simulink model "hw2_q3_part_two"  (R2022b)
settings: Solver=ode4  StartTime=0.0  StopTime=10.0  FixedStep=0.001  RelTol=1e-3
settings Model: Creator=gaura  LastModifiedBy=gaura

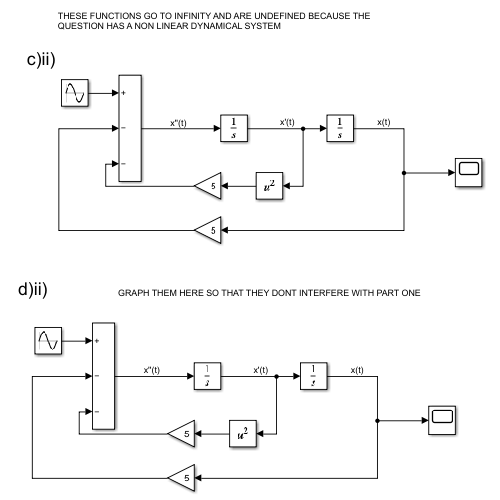
[thumbnail: Simulink's stored preview of the top-level diagram]
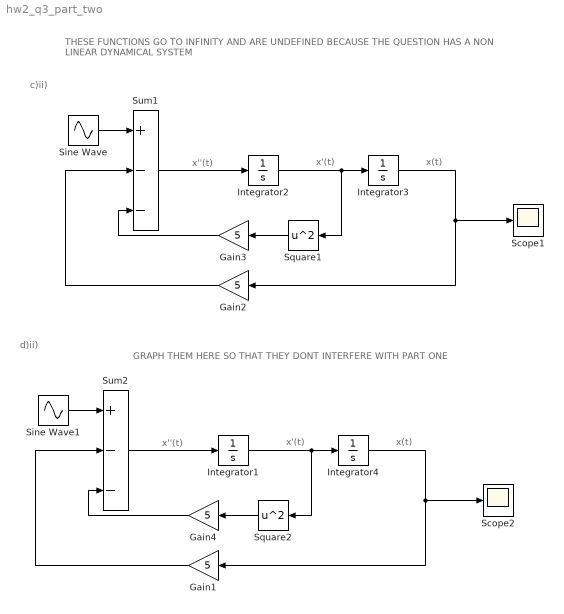
== system hw2_q3_part_two ==
  note: GRAPH THEM HERE SO THAT THEY DONT INTERFERE WITH PART ONE
  note: THESE FUNCTIONS GO TO INFINITY AND ARE UNDEFINED BECAUSE THE QUESTION HAS A NON LINEAR DYNAMICAL SYSTEM
  note: x'(t)
  note: x''(t)
  note: x(t)
  note: x(t)
  note: x''(t)
  note: x'(t)
  note: d)ii)
  note: c)ii)
  Gain{1..4} (4 alike) : Gain  Gain=5
  Integrator{1..4} (4 alike) : Integrator
  Scope1 : Scope
  Scope2 : Scope
  Sine Wave : Sin  Frequency=3  SampleTime=0
  Sine Wave1 : Sin  Amplitude=2  Frequency=3  SampleTime=0
  Square1 : Math  Operator=square
  Square2 : Math  Operator=square
  Sum1 : Sum  Inputs=+--
  Sum2 : Sum  Inputs=+--
  wires:
  Integrator2/1 -> Square1/1, Integrator3/1
  Sum1/1 -> Integrator2/1
  Gain3/1 -> Sum1/3
  Sine Wave/1 -> Sum1/1
  Square1/1 -> Gain3/1
  Integrator3/1 -> Gain2/1, Scope1/1
  Gain2/1 -> Sum1/2
  Gain1/1 -> Sum2/2
  Integrator4/1 -> Gain1/1, Scope2/1
  Integrator1/1 -> Square2/1, Integrator4/1
  Gain4/1 -> Sum2/3
  Sine Wave1/1 -> Sum2/1
  Square2/1 -> Gain4/1
  Sum2/1 -> Integrator1/1
